simulink model "programing_calculator"  (R2021b)
settings: Solver=VariableStepAuto  StartTime=0.0  StopTime=10.0  RelTol=1e-3
libraries: simulink x4
settings Model: Creator=midol  LastModifiedBy=midol

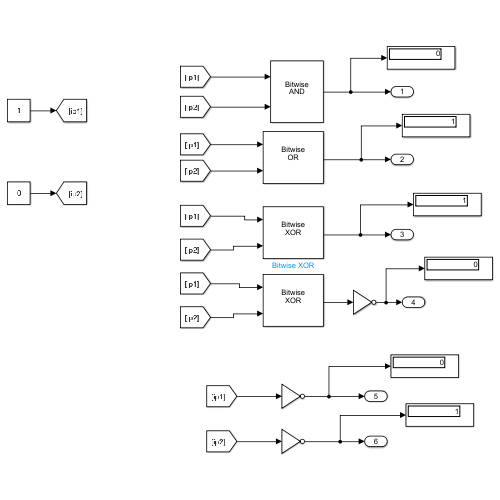
[thumbnail: Simulink's stored preview of the top-level diagram]
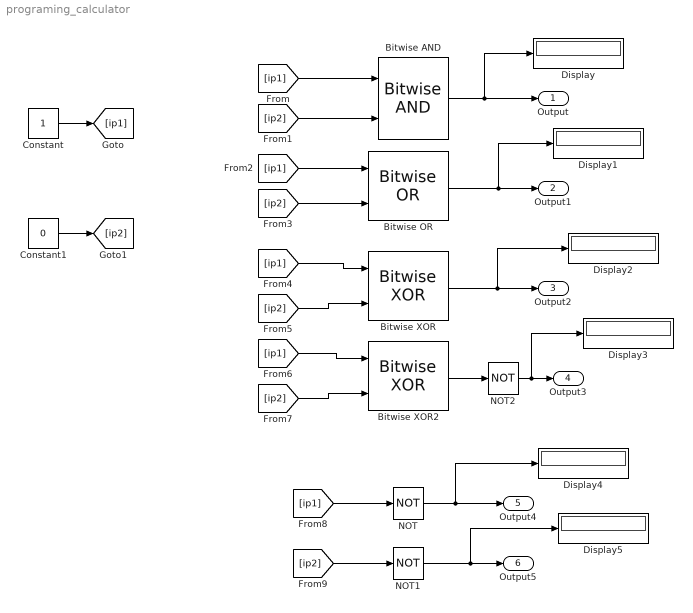
== system programing_calculator ==
  Bitwise AND : simulink/Logic and Bit Operations/Bitwise Operator  logicop=AND  UseBitMask=off  NumInputPorts=2  BitMask=bin2dec('11011001')  BitMaskRealWorld=Stored Integer
  Bitwise OR : simulink/Logic and Bit Operations/Bitwise Operator  logicop=OR  UseBitMask=off  NumInputPorts=2  BitMask=bin2dec('11011001')  BitMaskRealWorld=Stored Integer
  Bitwise XOR : simulink/Logic and Bit Operations/Bitwise Operator  logicop=XOR  UseBitMask=off  NumInputPorts=2  BitMask=bin2dec('11011001')  BitMaskRealWorld=Stored Integer
  Bitwise XOR2 : simulink/Logic and Bit Operations/Bitwise Operator  logicop=XOR  UseBitMask=off  NumInputPorts=2  BitMask=bin2dec('11011001')  BitMaskRealWorld=Stored Integer
  Constant : Constant  OutDataTypeStr=uint8
  Constant1 : Constant  Value=0  OutDataTypeStr=uint8
  Display{,1..5} (6 alike) : Display
  NOT : Logic  Operator=NOT  IconShape=distinctive  AllPortsSameDT=off  OutDataTypeStr=boolean
  NOT1 : Logic  Operator=NOT  IconShape=distinctive  AllPortsSameDT=off  OutDataTypeStr=boolean
  NOT2 : Logic  Operator=NOT  IconShape=distinctive  AllPortsSameDT=off  OutDataTypeStr=boolean
  Output : Outport
  Output1 : Outport  Port=2
  Output2 : Outport  Port=3
  Output3 : Outport  Port=4
  Output4 : Outport  Port=5
  Output5 : Outport  Port=6
  wires:
  [ip1] -> Bitwise AND/1
  [ip2] -> Bitwise AND/2
  [ip2] -> Bitwise OR/2
  [ip1] -> Bitwise OR/1
  [ip1] -> Bitwise XOR/1
  [ip2] -> Bitwise XOR/2
  [ip1] -> Bitwise XOR2/1
  Constant/1 -> [ip1]
  Constant1/1 -> [ip2]
  Bitwise AND/1 -> Display/1, Output/1
  Bitwise OR/1 -> Display1/1, Output1/1
  Bitwise XOR/1 -> Display2/1, Output2/1
  [ip1] -> NOT/1
  [ip2] -> NOT1/1
  NOT/1 -> Display4/1, Output4/1
  NOT1/1 -> Display5/1, Output5/1
  [ip2] -> Bitwise XOR2/2
  Bitwise XOR2/1 -> NOT2/1
  NOT2/1 -> Display3/1, Output3/1
